simulink library "Simulation_lib"  (R2023a)
settings: Solver=VariableStepAuto  StartTime=0.0  StopTime=10.0  RelTol=1e-3
libraries: $bdroot x14, fl_lib x8, nesl_utility x7, Math x5, ee_lib x3, sdl_lib x2, simulink_extras x1, vrlib x1
settings Model: Creator=FIRSTMentor  LastModifiedBy=FIRSTMentor

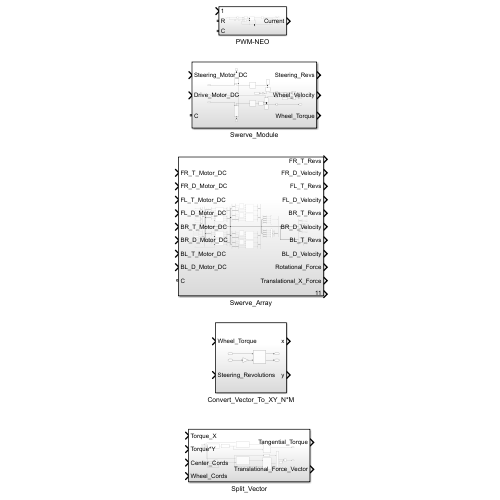
[thumbnail: Simulink's stored preview of the top-level diagram]
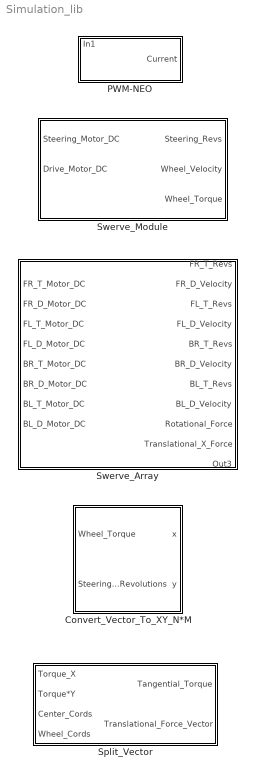
== system Simulation_lib ==
  Convert_Vector_To_XY_N*M : Subsystem
  PWM-NEO : Subsystem
  Split_Vector : Subsystem
  Swerve_Array : Subsystem
  Swerve_Module : Subsystem

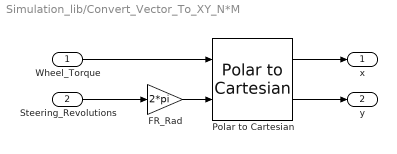
== system Simulation_lib/Convert_Vector_To_XY_N*M ==
  Wheel_Torque : Inport  OutDataTypeStr=double  Unit=N*m
  Steering_Revolutions : Inport  Port=2  OutDataTypeStr=double  Unit=rev  PortDimensions=1
  FR_Rad : Gain  Gain=2*pi
  Polar to Cartesian : simulink_extras/Transformations/Polar to Cartesian
  x : Outport  OutDataTypeStr=double  Unit=N*m  PortDimensions=1
  y : Outport  Port=2  OutDataTypeStr=double  Unit=N*m  PortDimensions=1
  wires:
  Steering_Revolutions/1 -> FR_Rad/1
  FR_Rad/1 -> Polar to Cartesian/2
  Polar to Cartesian/2 -> y/1
  Polar to Cartesian/1 -> x/1
  Wheel_Torque/1 -> Polar to Cartesian/1

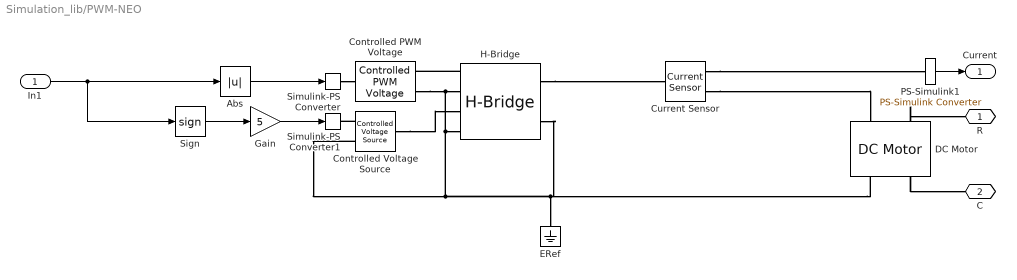
== system Simulation_lib/PWM-NEO ==
  In1 : Inport
  Abs : Abs  SaturateOnIntegerOverflow=off
  Controlled PWM Voltage : ee_lib/Integrated Circuits/Controlled PWM Voltage  F=4000 Hz  TD=0 s  pulse_width_offset=0 s  pulse_min=0 s  pwm_or_av=2  event_type=1  sample_time=5e-6 s  Vmin=0 V  Vmax=5 V  Vm=5 V  u_min=0  u_max=1
      settings: InternalSimscapePortConfiguration="{\"Bottom\":[],\"Left\":[{\"id\":\"u\",\"label\":\"u\",\"type\":\"input\"}],\"Right\":[{\"id\":\"p2\",\"label\":\"PWM\",\"type\":\"foundation.electrical.electrical\"},{\"id\":\"n2\",\"label\":\"REF\",\"type\":\"foundation.electrical.electrical\"}],\"Top\":[]}"
  Controlled Voltage Source : fl_lib/Electrical/Electrical Sources/Controlled Voltage Source
  Current Sensor : fl_lib/Electrical/Electrical Sensors/Current Sensor
  DC Motor : ee_lib/Electromechanical/Brushed Motors/DC Motor  field_option=ee.enum.field_option.pm  Rf=100 Ohm  Lf=1 H  Laf=0.15 H  If0=0 A  parameterization=3  Ra=3.38 Ohm  La=0.01 H  emf_or_torque=1  Kv=0.029 V/(rad/s)  Ki=6.876e-04 N*m/A  T_stall=0.1 N*m  w_max=5700 rpm  w_rated=2910 rpm  P_rated=500 W  V_rated=12 V  lam_param=ee.enum.lam_param.current  i_noload=1.7 A  V_i_noload=12 V  J=0.0002 kg*m^2  lam=0.5e-5 N*m/(rad/s)  speed0=0 rpm  enable_fault_armature=simscape.enum.onoff.off  rev_faulted=1 / 3  G_faulted_armature=1e-5 S  fault_trigger_armature=ee.enum.faults.faultTrigger.temporal  t_fault_armature=1 s  max_permissible_current_armature=inf A  t_fail_on_current_armature=1 s  enable_fault_field=simscape.enum.onoff.off  G_faulted_field=1e-5 S  fault_trigger_field=ee.enum.faults.faultTrigger.temporal  t_fault_field=1 s  max_permissible_current_field=inf A  t_fail_on_current_field=1 s  fault_action=simscape.enum.assert.action.none  alpha=3.93e-3 1/K  Tmeas=25 degC  thermal_mass=100 J/K  initial_temperature=25 degC
  ERef : fl_lib/Electrical/Electrical Elements/Electrical Reference
  Gain : Gain  Gain=5
  H-Bridge : ee_lib/Semiconductors & Converters/Converters/H-Bridge  supply_ports=ee.enum.supply_ports.hidesupply  pwm_or_av=2  regenerative_braking_mode=2  discontinuous=0  freewheeling_mode=1  Rload=3.38+0.1 Ohm  Lload=1e-5 H  F=4 kHz  Venable=2.5 V  Vmax=5 V  Vreverse=2.5 V  Vbrake=2.5 V  Vm=12 V  Ron=0.1 Ohm  Don=0.1 Ohm  Goff=1e-6 S  Tmeas=298.15 K  Ron2=0.1 Ohm  Don2=0.05 Ohm  Tmeas2=398.15 K  thermal_mass=100 J/K  initial_temperature=298.15 K
  PS-Simulink1 : nesl_utility/PS-Simulink Converter  PhysicalDomain=network_engine_domain  SubClassName=ps_output  LeftPortType=input  RightPortType=output  PseudoPeriodic=off  Frequencies=[]  VectorFormat=1-D array  Unit=A  AffineConversion=off
  Sign : Signum
  Simulink-PS Converter : nesl_utility/Simulink-PS Converter  PhysicalDomain=network_engine_domain  SubClassName=ps_input  LeftPortType=input  RightPortType=output  PseudoPeriodic=off  Frequencies=[]  NoiseDistribution=none  NoiseParameters=[]  Unit=1  AffineConversion=off  FilteringAndDerivatives=provide  SimscapeFilterOrder=1  InputFilterTimeConstant=0.001  UdotUserProvided=0
  Simulink-PS Converter1 : nesl_utility/Simulink-PS Converter  PhysicalDomain=network_engine_domain  SubClassName=ps_input  LeftPortType=input  RightPortType=output  PseudoPeriodic=off  Frequencies=[]  NoiseDistribution=none  NoiseParameters=[]  Unit=1  AffineConversion=off  FilteringAndDerivatives=zero  SimscapeFilterOrder=1  InputFilterTimeConstant=0.001  UdotUserProvided=0
  R : PMIOPort  Side=Left
  C : PMIOPort  Port=2  Side=Left
  Current : Outport
  wires:
  PS-Simulink1/1 -> Current/1
  Abs/1 -> Simulink-PS Converter/1
  In1/1 -> Sign/1, Abs/1
  Sign/1 -> Gain/1
  Gain/1 -> Simulink-PS Converter1/1
  connections:
  Current Sensor/RConn1 -- PS-Simulink1/LConn1
  H-Bridge/RConn1 -- Current Sensor/LConn1
  H-Bridge/LConn1 -- Controlled PWM Voltage/RConn1
  Simulink-PS Converter/RConn1 -- Controlled PWM Voltage/LConn1
  DC Motor/RConn2 -- C/RConn1
  DC Motor/LConn2 -- R/RConn1
  Current Sensor/RConn2 -- DC Motor/LConn1
  H-Bridge/LConn4 -- Controlled Voltage Source/RConn2 -- DC Motor/RConn1 -- H-Bridge/RConn2 -- ERef/LConn1 -- H-Bridge/LConn2 -- Controlled PWM Voltage/RConn2
  Controlled Voltage Source/LConn1 -- H-Bridge/LConn3
  Controlled Voltage Source/RConn1 -- Simulink-PS Converter1/RConn1

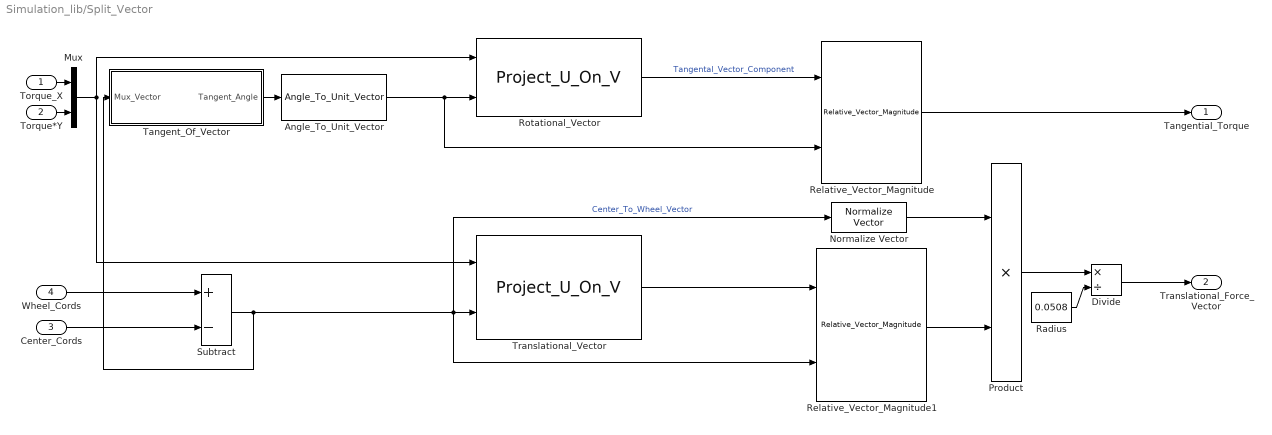
== system Simulation_lib/Split_Vector ==
  Torque_X : Inport  OutDataTypeStr=double  Unit=N*m  PortDimensions=1
  Torque*Y : Inport  Port=2  OutDataTypeStr=double  Unit=N*m  PortDimensions=1
  Center_Cords : Inport  Port=3  OutDataTypeStr=double  Unit=m  PortDimensions=2
  Wheel_Cords : Inport  Port=4  OutDataTypeStr=double  Unit=m  PortDimensions=2
  Angle_To_Unit_Vector : Math/Angle_To_Unit_Vector  SystemSampleTime=-1  VariantActivationTime=update diagram  Latency=0  AutoFrameSizeCalculation=off
  Divide : Product  Inputs=*/
  Mux : Mux  Inputs=2
  Normalize Vector : vrlib/Utilities/Normalize Vector  maxzero=0
  Product : Product
  Radius : Constant  Value=0.0508
  Relative_Vector_Magnitude : Math/Relative_Vector_Magnitude  SystemSampleTime=-1  VariantActivationTime=update diagram  Latency=0  AutoFrameSizeCalculation=off
  Relative_Vector_Magnitude1 : Math/Relative_Vector_Magnitude  SystemSampleTime=-1  VariantActivationTime=update diagram  Latency=0  AutoFrameSizeCalculation=off
  Rotational_Vector : Math/Project_U_On_V  SystemSampleTime=-1  VariantActivationTime=update diagram  Latency=0  AutoFrameSizeCalculation=off
  Subtract : Sum  Inputs=+-
  Tangent_Of_Vector : Subsystem
  Translational_Vector : Math/Project_U_On_V  SystemSampleTime=-1  VariantActivationTime=update diagram  Latency=0  AutoFrameSizeCalculation=off
  Tangential_Torque : Outport  OutDataTypeStr=double  Unit=N*m
  Translational_Force_Vector : Outport  Port=2  OutDataTypeStr=double  Unit=N  PortDimensions=2
  wires:
  Torque_X/1 -> Mux/1
  Torque*Y/1 -> Mux/2
  Mux/1 -> Translational_Vector/1, Rotational_Vector/1
  Tangent_Of_Vector/1(Tangent_Angle) -> Angle_To_Unit_Vector/1
  Center_Cords/1 -> Subtract/2
  Subtract/1 -> Tangent_Of_Vector/1(Mux_Vector), Relative_Vector_Magnitude1/2, Normalize Vector/1, Translational_Vector/2  "Center_To_Wheel_Vector"
  Wheel_Cords/1 -> Subtract/1
  Rotational_Vector/1 -> Relative_Vector_Magnitude/1  "Tangental_Vector_Component"
  Relative_Vector_Magnitude/1 -> Tangential_Torque/1
  Relative_Vector_Magnitude1/1 -> Product/2
  Translational_Vector/1 -> Relative_Vector_Magnitude1/1
  Normalize Vector/1 -> Product/1
  Product/1 -> Divide/1
  Angle_To_Unit_Vector/1 -> Rotational_Vector/2, Relative_Vector_Magnitude/2
  Divide/1 -> Translational_Force_Vector/1
  Radius/1 -> Divide/2

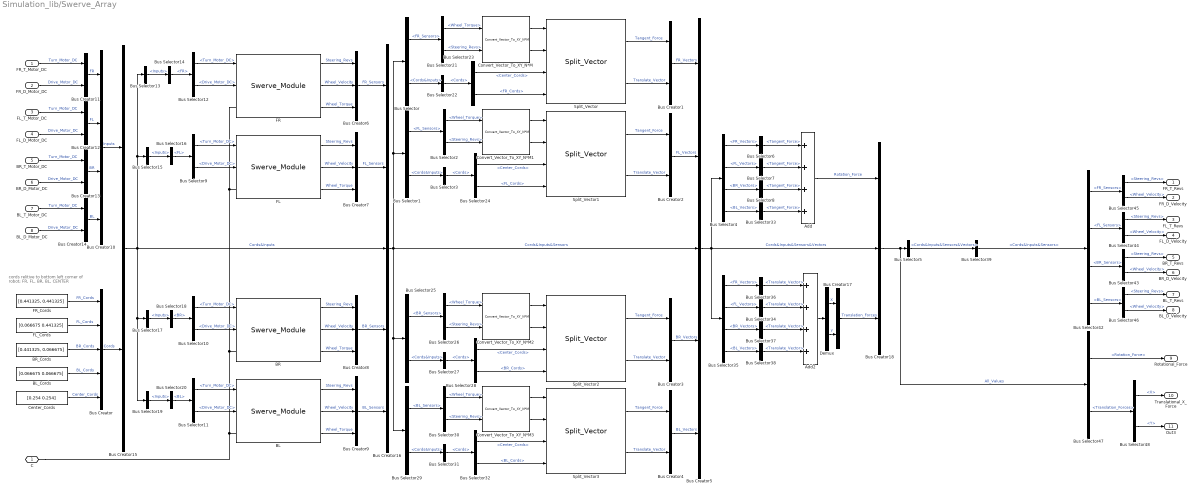
== system Simulation_lib/Swerve_Array ==
  note: cords relitive to bottom left corner of robot; FR, FL, BR, BL, CENTER
  FR_T_Motor_DC : Inport
  FR_D_Motor_DC : Inport  Port=2
  FL_T_Motor_DC : Inport  Port=3
  FL_D_Motor_DC : Inport  Port=4
  BR_T_Motor_DC : Inport  Port=5
  BR_D_Motor_DC : Inport  Port=6
  BL_T_Motor_DC : Inport  Port=7
  BL_D_Motor_DC : Inport  Port=8
  Add : Sum  Inputs=4
  Add2 : Sum  Inputs=4
  BL : $bdroot/Swerve_Module  SystemSampleTime=-1  VariantActivationTime=update diagram  Latency=0  AutoFrameSizeCalculation=off
  BL_Cords : Constant  Value=[0.066675 0.066675]
  BR : $bdroot/Swerve_Module  SystemSampleTime=-1  VariantActivationTime=update diagram  Latency=0  AutoFrameSizeCalculation=off
  BR_Cords : Constant  Value=[0.441325, 0.066675]
  Bus Creator : BusCreator  Inputs=5
  Bus Creator{1..4,11..15,17} (10 alike) : BusCreator  Inputs=2
  Bus Creator10 : BusCreator  Inputs=4
  Bus Creator16 : BusCreator  Inputs=5
  Bus Creator{6..9,18} (5 alike) : BusCreator  Inputs=3
  Bus Creator5 : BusCreator  Inputs=5
  Bus Selector : BusSelector  OutputSignals=FR_Sensors,Cords&Inputs
  Bus Selector1 : BusSelector  OutputSignals=FL_Sensors,Cords&Inputs
  Bus Selector{9..12} (4 alike) : BusSelector  OutputSignals=Turn_Motor_DC,Drive_Motor_DC
  Bus Selector{13,15,17,19} (4 alike) : BusSelector  OutputSignals=Inputs
  Bus Selector14 : BusSelector  OutputSignals=FR
  Bus Selector16 : BusSelector  OutputSignals=FL
  Bus Selector18 : BusSelector  OutputSignals=BR
  Bus Selector{2,21,26,30} (4 alike) : BusSelector  OutputSignals=Wheel_Torque,Steering_Revs
  Bus Selector20 : BusSelector  OutputSignals=BL
  Bus Selector{3,22,27,31} (4 alike) : BusSelector  OutputSignals=Cords
  Bus Selector23 : BusSelector  OutputSignals=Center_Cords,FR_Cords
  Bus Selector24 : BusSelector  OutputSignals=Center_Cords,FL_Cords
  Bus Selector25 : BusSelector  OutputSignals=BR_Sensors,Cords&Inputs
  Bus Selector28 : BusSelector  OutputSignals=Center_Cords,BR_Cords
  Bus Selector29 : BusSelector  OutputSignals=BL_Sensors,Cords&Inputs
  Bus Selector32 : BusSelector  OutputSignals=Center_Cords,BL_Cords
  Bus Selector{6..8,33} (4 alike) : BusSelector  OutputSignals=Tangent_Force
  Bus Selector{34,36..38} (4 alike) : BusSelector  OutputSignals=Translate_Vector
  Bus Selector35 : BusSelector  OutputSignals=FR_Vectors,FL_Vectors,BR_Vectors,BL_Vectors
  Bus Selector39 : BusSelector  OutputSignals=Cords&Inputs&Sensors
  Bus Selector4 : BusSelector  OutputSignals=FR_Vectors,FL_Vectors,BR_Vectors,BL_Vectors
  Bus Selector42 : BusSelector  OutputSignals=FR_Sensors,FL_Sensors,BR_Sensors,BL_Sensors
  Bus Selector{43..46} (4 alike) : BusSelector  OutputSignals=Steering_Revs,Wheel_Velocity
  Bus Selector47 : BusSelector  OutputSignals=Rotation_Force,Translation_Forces
  Bus Selector48 : BusSelector  OutputSignals=X,Y
  Bus Selector5 : BusSelector  OutputSignals=Cords&Inputs&Sensors&Vectors
  Center_Cords : Constant  Value=[0.254 0.254]
  Convert_Vector_To_XY_N*M{,1..3} (4 alike) : $bdroot/Convert_Vector_To_XY_N*M  SystemSampleTime=-1  VariantActivationTime=update diagram  Latency=0  AutoFrameSizeCalculation=off
  Demux : Demux  Outputs=2
  FL : $bdroot/Swerve_Module  SystemSampleTime=-1  VariantActivationTime=update diagram  Latency=0  AutoFrameSizeCalculation=off
  FL_Cords : Constant  Value=[0.066675 0.441325]
  FR : $bdroot/Swerve_Module  SystemSampleTime=-1  VariantActivationTime=update diagram  Latency=0  AutoFrameSizeCalculation=off
  FR_Cords : Constant  Value=[0.441325, 0.441325]
  Split_Vector{,1..3} (4 alike) : $bdroot/Split_Vector  SystemSampleTime=-1  VariantActivationTime=update diagram  Latency=0  AutoFrameSizeCalculation=off
  C : PMIOPort  Side=Left
  FR_T_Revs : Outport
  FR_D_Velocity : Outport  Port=2
  FL_T_Revs : Outport  Port=3
  FL_D_Velocity : Outport  Port=4
  BR_T_Revs : Outport  Port=5
  BR_D_Velocity : Outport  Port=6
  BL_T_Revs : Outport  Port=7
  BL_D_Velocity : Outport  Port=8
  Rotational_Force : Outport  Port=9
  Translational_X_Force : Outport  Port=10
  Out3 : Outport  Port=11
  wires:
  FR_Cords/1 -> Bus Creator/1  "FR_Cords"
  FL_Cords/1 -> Bus Creator/2  "FL_Cords"
  BR_Cords/1 -> Bus Creator/3  "BR_Cords"
  BL_Cords/1 -> Bus Creator/4  "BL_Cords"
  Center_Cords/1 -> Bus Creator/5  "Center_Cords"
  Convert_Vector_To_XY_N*M/1 -> Split_Vector/1
  Convert_Vector_To_XY_N*M/2 -> Split_Vector/2
  Convert_Vector_To_XY_N*M1/1 -> Split_Vector1/1
  Convert_Vector_To_XY_N*M1/2 -> Split_Vector1/2
  Convert_Vector_To_XY_N*M2/1 -> Split_Vector2/1
  Convert_Vector_To_XY_N*M2/2 -> Split_Vector2/2
  Convert_Vector_To_XY_N*M3/1 -> Split_Vector3/1
  Convert_Vector_To_XY_N*M3/2 -> Split_Vector3/2
  Split_Vector/1 -> Bus Creator1/1  "Tangent_Force"
  Split_Vector/2 -> Bus Creator1/2  "Translate_Vector"
  Split_Vector1/2 -> Bus Creator2/2  "Translate_Vector"
  Split_Vector1/1 -> Bus Creator2/1  "Tangent_Force"
  Split_Vector2/1 -> Bus Creator3/1  "Tangent_Force"
  Split_Vector2/2 -> Bus Creator3/2  "Translate_Vector"
  Split_Vector3/2 -> Bus Creator4/2  "Translate_Vector"
  Split_Vector3/1 -> Bus Creator4/1  "Tangent_Force"
  Bus Creator1/1 -> Bus Creator5/1  "FR_Vectors"
  Bus Creator2/1 -> Bus Creator5/2  "FL_Vectors"
  Bus Creator3/1 -> Bus Creator5/4  "BR_Vectors"
  Bus Creator4/1 -> Bus Creator5/5  "BL_Vectors"
  FR/2 -> Bus Creator6/2  "Wheel_Velocity"
  FR/1 -> Bus Creator6/1  "Steering_Revs"
  FR/3 -> Bus Creator6/3  "Wheel_Torque"
  FL/1 -> Bus Creator7/1  "Steering_Revs"
  FL/2 -> Bus Creator7/2  "Wheel_Velocity"
  FL/3 -> Bus Creator7/3  "Wheel_Torque"
  BL/1 -> Bus Creator9/1  "Steering_Revs"
  BL/2 -> Bus Creator9/2  "Wheel_Velocity"
  BL/3 -> Bus Creator9/3  "Wheel_Torque"
  BR/3 -> Bus Creator8/3  "Wheel_Torque"
  BR/2 -> Bus Creator8/2  "Wheel_Velocity"
  BR/1 -> Bus Creator8/1  "Steering_Revs"
  FR_T_Motor_DC/1 -> Bus Creator11/1  "Turn_Motor_DC"
  FR_D_Motor_DC/1 -> Bus Creator11/2  "Drive_Motor_DC"
  FL_T_Motor_DC/1 -> Bus Creator12/1  "Turn_Motor_DC"
  FL_D_Motor_DC/1 -> Bus Creator12/2  "Drive_Motor_DC"
  BR_T_Motor_DC/1 -> Bus Creator13/1  "Turn_Motor_DC"
  BR_D_Motor_DC/1 -> Bus Creator13/2  "Drive_Motor_DC"
  BL_T_Motor_DC/1 -> Bus Creator14/1  "Turn_Motor_DC"
  BL_D_Motor_DC/1 -> Bus Creator14/2  "Drive_Motor_DC"
  Bus Creator12/1 -> Bus Creator10/2  "FL"
  Bus Creator11/1 -> Bus Creator10/1  "FR"
  Bus Creator13/1 -> Bus Creator10/3  "BR"
  Bus Creator14/1 -> Bus Creator10/4  "BL"
  Bus Creator10/1 -> Bus Creator15/1  "Inputs"
  Bus Creator/1 -> Bus Creator15/2  "Cords"
  Bus Creator15/1 -> Bus Selector19/1, Bus Selector17/1, Bus Creator16/3, Bus Selector13/1, Bus Selector15/1  "Cords&Inputs"
  Bus Selector9/1 -> FL/1  "<Turn_Motor_DC>"
  Bus Selector9/2 -> FL/2  "<Drive_Motor_DC>"
  Bus Selector10/1 -> BR/1  "<Turn_Motor_DC>"
  Bus Selector10/2 -> BR/2  "<Drive_Motor_DC>"
  Bus Selector11/1 -> BL/1  "<Turn_Motor_DC>"
  Bus Selector11/2 -> BL/2  "<Drive_Motor_DC>"
  Bus Selector12/1 -> FR/1  "<Turn_Motor_DC>"
  Bus Selector12/2 -> FR/2  "<Drive_Motor_DC>"
  Bus Selector13/1 -> Bus Selector14/1  "<Inputs>"
  Bus Selector14/1 -> Bus Selector12/1  "<FR>"
  Bus Selector15/1 -> Bus Selector16/1  "<Inputs>"
  Bus Selector16/1 -> Bus Selector9/1  "<FL>"
  Bus Selector17/1 -> Bus Selector18/1  "<Inputs>"
  Bus Selector18/1 -> Bus Selector10/1  "<BR>"
  Bus Selector19/1 -> Bus Selector20/1  "<Inputs>"
  Bus Selector20/1 -> Bus Selector11/1  "<BL>"
  Bus Creator6/1 -> Bus Creator16/1  "FR_Sensors"
  Bus Creator7/1 -> Bus Creator16/2  "FL_Sensors"
  Bus Creator9/1 -> Bus Creator16/5  "BL_Sensors"
  Bus Creator8/1 -> Bus Creator16/4  "BR_Sensors"
  Bus Creator16/1 -> Bus Selector/1, Bus Selector1/1, Bus Creator5/3, Bus Selector29/1, Bus Selector25/1  "Cords&Inputs&Sensors"
  Bus Selector/1 -> Bus Selector21/1  "<FR_Sensors>"
  Bus Selector21/1 -> Convert_Vector_To_XY_N*M/1  "<Wheel_Torque>"
  Bus Selector21/2 -> Convert_Vector_To_XY_N*M/2  "<Steering_Revs>"
  Bus Selector/2 -> Bus Selector22/1  "<Cords&Inputs>"
  Bus Selector22/1 -> Bus Selector23/1  "<Cords>"
  Bus Selector23/1 -> Split_Vector/3  "<Center_Cords>"
  Bus Selector23/2 -> Split_Vector/4  "<FR_Cords>"
  Bus Selector2/1 -> Convert_Vector_To_XY_N*M1/1  "<Wheel_Torque>"
  Bus Selector3/1 -> Bus Selector24/1  "<Cords>"
  Bus Selector24/2 -> Split_Vector1/4  "<FL_Cords>"
  Bus Selector1/2 -> Bus Selector3/1  "<Cords&Inputs>"
  Bus Selector1/1 -> Bus Selector2/1  "<FL_Sensors>"
  Bus Selector2/2 -> Convert_Vector_To_XY_N*M1/2  "<Steering_Revs>"
  Bus Selector24/1 -> Split_Vector1/3  "<Center_Cords>"
  Bus Selector26/1 -> Convert_Vector_To_XY_N*M2/1  "<Wheel_Torque>"
  Bus Selector27/1 -> Bus Selector28/1  "<Cords>"
  Bus Selector28/2 -> Split_Vector2/4  "<BR_Cords>"
  Bus Selector25/2 -> Bus Selector27/1  "<Cords&Inputs>"
  Bus Selector25/1 -> Bus Selector26/1  "<BR_Sensors>"
  Bus Selector26/2 -> Convert_Vector_To_XY_N*M2/2  "<Steering_Revs>"
  Bus Selector28/1 -> Split_Vector2/3  "<Center_Cords>"
  Bus Selector30/1 -> Convert_Vector_To_XY_N*M3/1  "<Wheel_Torque>"
  Bus Selector31/1 -> Bus Selector32/1  "<Cords>"
  Bus Selector32/2 -> Split_Vector3/4  "<BL_Cords>"
  Bus Selector29/2 -> Bus Selector31/1  "<Cords&Inputs>"
  Bus Selector29/1 -> Bus Selector30/1  "<BL_Sensors>"
  Bus Selector30/2 -> Convert_Vector_To_XY_N*M3/2  "<Steering_Revs>"
  Bus Selector32/1 -> Split_Vector3/3  "<Center_Cords>"
  Bus Selector4/1 -> Bus Selector6/1  "<FR_Vectors>"
  Bus Selector4/2 -> Bus Selector7/1  "<FL_Vectors>"
  Bus Selector4/3 -> Bus Selector8/1  "<BR_Vectors>"
  Bus Selector4/4 -> Bus Selector33/1  "<BL_Vectors>"
  Bus Selector6/1 -> Add/1  "<Tangent_Force>"
  Bus Selector7/1 -> Add/2  "<Tangent_Force>"
  Bus Selector8/1 -> Add/3  "<Tangent_Force>"
  Bus Selector33/1 -> Add/4  "<Tangent_Force>"
  Add/1 -> Bus Creator18/1  "Rotation_Force"
  Bus Creator5/1 -> Bus Selector4/1, Bus Creator18/2, Bus Selector35/1  "Cords&Inputs&Sensors&Vectors"
  Bus Selector38/1 -> Add2/4  "<Translate_Vector>"
  Bus Selector35/4 -> Bus Selector38/1  "<BL_Vectors>"
  Demux/1 -> Bus Creator17/1  "X"
  Bus Selector34/1 -> Add2/2  "<Translate_Vector>"
  Demux/2 -> Bus Creator17/2  "Y"
  Add2/1 -> Demux/1
  Bus Selector35/3 -> Bus Selector37/1  "<BR_Vectors>"
  Bus Selector35/2 -> Bus Selector34/1  "<FL_Vectors>"
  Bus Selector37/1 -> Add2/3  "<Translate_Vector>"
  Bus Selector36/1 -> Add2/1  "<Translate_Vector>"
  Bus Selector35/1 -> Bus Selector36/1  "<FR_Vectors>"
  Bus Creator17/1 -> Bus Creator18/3  "Translation_Forces"
  Bus Creator18/1 -> Bus Selector5/1, Bus Selector47/1  "All_Values"
  Bus Selector5/1 -> Bus Selector39/1  "<Cords&Inputs&Sensors&Vectors>"
  Bus Selector39/1 -> Bus Selector42/1  "<Cords&Inputs&Sensors>"
  Bus Selector42/4 -> Bus Selector46/1  "<BL_Sensors>"
  Bus Selector46/1 -> BL_T_Revs/1  "<Steering_Revs>"
  Bus Selector46/2 -> BL_D_Velocity/1  "<Wheel_Velocity>"
  Bus Selector43/1 -> BR_T_Revs/1  "<Steering_Revs>"
  Bus Selector43/2 -> BR_D_Velocity/1  "<Wheel_Velocity>"
  Bus Selector42/3 -> Bus Selector43/1  "<BR_Sensors>"
  Bus Selector44/1 -> FL_T_Revs/1  "<Steering_Revs>"
  Bus Selector44/2 -> FL_D_Velocity/1  "<Wheel_Velocity>"
  Bus Selector42/2 -> Bus Selector44/1  "<FL_Sensors>"
  Bus Selector45/1 -> FR_T_Revs/1  "<Steering_Revs>"
  Bus Selector45/2 -> FR_D_Velocity/1  "<Wheel_Velocity>"
  Bus Selector42/1 -> Bus Selector45/1  "<FR_Sensors>"
  Bus Selector47/1 -> Rotational_Force/1  "<Rotation_Force>"
  Bus Selector47/2 -> Bus Selector48/1  "<Translation_Forces>"
  Bus Selector48/2 -> Out3/1  "<Y>"
  Bus Selector48/1 -> Translational_X_Force/1  "<X>"
  connections:
  BR/LConn1 -- C/RConn1 -- BL/LConn1 -- FR/LConn1 -- FL/LConn1

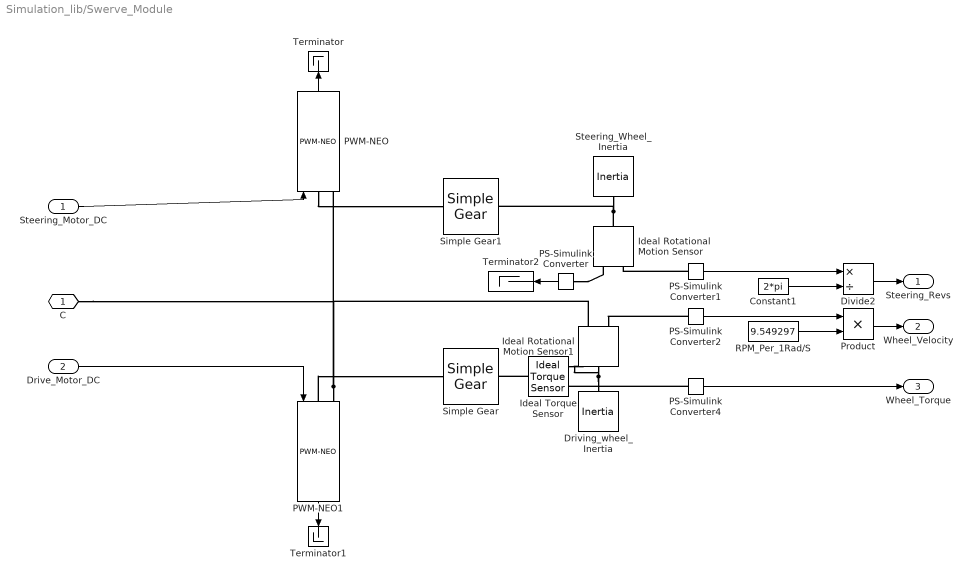
== system Simulation_lib/Swerve_Module ==
  Steering_Motor_DC : Inport
  Drive_Motor_DC : Inport  Port=2
  Constant1 : Constant  Value=2*pi
  Divide2 : Product  Inputs=*/
  Driving_wheel_Inertia : fl_lib/Mechanical/Rotational Elements/Inertia  inertia=1.315 lbm*in^2  num_ports=foundation.enum.numPorts2.one  w_specify=off  w_priority=High  w=0 rad/s  w_nominal_specify=off  w_nominal_unit=rad/s  w_nominal_value=1  t_specify=off  t_priority=None  t=0 N*m  t_nominal_specify=off  t_nominal_unit=N*m  t_nominal_value=1
  Ideal Rotational Motion Sensor : fl_lib/Mechanical/Mechanical Sensors/Ideal Rotational Motion Sensor  reference=foundation.enum.MeasurementReference.absolute  acceleration_port=false  velocity_port=true  position_port=true  wrap_angle=false  offset=0 rad
      settings: InternalSimscapePortConfiguration="{\"Bottom\":[],\"Left\":[{\"id\":\"R\",\"label\":\"R\",\"type\":\"foundation.mechanical.rotational.rotational\"}],\"Right\":[{\"id\":\"W\",\"label\":\"W\",\"type\":\"output\"},{\"id\":\"A\",\"label\":\"A\",\"type\":\"output\"}],\"Top\":[]}"
  Ideal Rotational Motion Sensor1 : fl_lib/Mechanical/Mechanical Sensors/Ideal Rotational Motion Sensor  reference=foundation.enum.MeasurementReference.difference  acceleration_port=false  velocity_port=true  position_port=false  wrap_angle=false  offset=0 rad
      settings: InternalSimscapePortConfiguration="{\"Bottom\":[],\"Left\":[{\"id\":\"R\",\"label\":\"R\",\"type\":\"foundation.mechanical.rotational.rotational\"}],\"Right\":[{\"id\":\"C\",\"label\":\"C\",\"type\":\"foundation.mechanical.rotational.rotational\"},{\"id\":\"W\",\"label\":\"W\",\"type\":\"output\"}],\"Top\":[]}"
  Ideal Torque Sensor : fl_lib/Mechanical/Mechanical Sensors/Ideal Torque Sensor
  PS-Simulink Converter : nesl_utility/PS-Simulink Converter  PhysicalDomain=network_engine_domain  SubClassName=ps_output  LeftPortType=input  RightPortType=output  PseudoPeriodic=off  Frequencies=[]  VectorFormat=inherit  Unit=inherit  AffineConversion=off
  PS-Simulink Converter1 : nesl_utility/PS-Simulink Converter  PhysicalDomain=network_engine_domain  SubClassName=ps_output  LeftPortType=input  RightPortType=output  PseudoPeriodic=off  Frequencies=[]  VectorFormat=inherit  Unit=inherit  AffineConversion=off
  PS-Simulink Converter2 : nesl_utility/PS-Simulink Converter  PhysicalDomain=network_engine_domain  SubClassName=ps_output  LeftPortType=input  RightPortType=output  PseudoPeriodic=off  Frequencies=[]  VectorFormat=inherit  Unit=rad/s  AffineConversion=off
  PS-Simulink Converter4 : nesl_utility/PS-Simulink Converter  PhysicalDomain=network_engine_domain  SubClassName=ps_output  LeftPortType=input  RightPortType=output  PseudoPeriodic=off  Frequencies=[]  VectorFormat=inherit  Unit=inherit  AffineConversion=off
  PWM-NEO : $bdroot/PWM-NEO  SystemSampleTime=-1  VariantActivationTime=update diagram  Latency=0  AutoFrameSizeCalculation=off
  PWM-NEO1 : $bdroot/PWM-NEO  SystemSampleTime=-1  VariantActivationTime=update diagram  Latency=0  AutoFrameSizeCalculation=off
  Product : Product
  RPM_Per_1Rad/S : Constant  Value=9.549297
  Simple Gear : sdl_lib/Gears/Simple Gear  ratio=8.14  rotation_direction=sdl.enum.shaftOutputDirection.opposite  friction_model=sdl.enum.gear_efficiencies_load.off  T_noload=0.1 N*m  T_nom=5 N*m  efficiency_nom=0.8  efficiency=0.8  temperature_TLU=[280, 300, 320] K  load_TLU=[1, 5, 10] N*m  efficiency_TLU=[.95, .9, .85]  efficiency_TLU2=[.85, .8, .75; .95, .9, .85; .85, .8, .7]  w_thr=0.01 rad/s  pwr_thr=0.001 W  enable_backlash=false  hardstop_model=simscape.enum.hardstop.smooth  backlash_distance=1e-3 mm  r_base=0.1 m  transition=1e-4 mm  backlash_stiffness=1e6 N/m  backlash_damping=1e3 N*s/m  coeff_rest=0.7  v_tol=0.001 m/s  f_tol=0.001 N  mu_visc=[0, 0] N*m*s/rad  enable_faults=simscape.enum.onoff.off  efficiency_fault=0.05  external_fault=simscape.enum.onoff.off  temporal_fault=simscape.enum.onoff.off  fault_time=5 s  fault_angles=pi / 12 rad  report_fault=simscape.enum.assert.action.none  thermal_mass=50 J/K  temperature_specify=off  temperature_priority=High  temperature=300 K  temperature_nominal_specify=off  temperature_nominal_unit=K  temperature_nominal_value=1  x_backlash_specify=off  x_backlash_priority=None  x_backlash=0 mm  x_backlash_nominal_specify=off  x_backlash_nominal_unit=mm  x_backlash_nominal_value=1  f_hardstop_specify=off  f_hardstop_priority=None  f_hardstop=0 N  f_hardstop_nominal_specify=off  f_hardstop_nominal_unit=N  f_hardstop_nominal_value=1  v_backlash_specify=off  v_backlash_priority=None  v_backlash=0 m/s  v_backlash_nominal_specify=off  v_backlash_nominal_unit=m/s  v_backlash_nominal_value=1
  Simple Gear1 : sdl_lib/Gears/Simple Gear  ratio=150/7  rotation_direction=sdl.enum.shaftOutputDirection.opposite  friction_model=sdl.enum.gear_efficiencies_load.off  T_noload=0.1 N*m  T_nom=5 N*m  efficiency_nom=0.8  efficiency=0.8  temperature_TLU=[280, 300, 320] K  load_TLU=[1, 5, 10] N*m  efficiency_TLU=[.95, .9, .85]  efficiency_TLU2=[.85, .8, .75; .95, .9, .85; .85, .8, .7]  w_thr=0.01 rad/s  pwr_thr=0.001 W  enable_backlash=false  hardstop_model=simscape.enum.hardstop.smooth  backlash_distance=1e-3 mm  r_base=0.1 m  transition=1e-4 mm  backlash_stiffness=1e6 N/m  backlash_damping=1e3 N*s/m  coeff_rest=0.7  v_tol=0.001 m/s  f_tol=0.001 N  mu_visc=[0, 0] N*m*s/rad  enable_faults=simscape.enum.onoff.off  efficiency_fault=0.05  external_fault=simscape.enum.onoff.off  temporal_fault=simscape.enum.onoff.off  fault_time=5 s  fault_angles=pi / 12 rad  report_fault=simscape.enum.assert.action.none  thermal_mass=50 J/K  temperature_specify=off  temperature_priority=High  temperature=300 K  temperature_nominal_specify=off  temperature_nominal_unit=K  temperature_nominal_value=1  x_backlash_specify=off  x_backlash_priority=None  x_backlash=0 mm  x_backlash_nominal_specify=off  x_backlash_nominal_unit=mm  x_backlash_nominal_value=1  f_hardstop_specify=off  f_hardstop_priority=None  f_hardstop=0 N  f_hardstop_nominal_specify=off  f_hardstop_nominal_unit=N  f_hardstop_nominal_value=1  v_backlash_specify=off  v_backlash_priority=None  v_backlash=0 m/s  v_backlash_nominal_specify=off  v_backlash_nominal_unit=m/s  v_backlash_nominal_value=1
  Steering_Wheel_Inertia : fl_lib/Mechanical/Rotational Elements/Inertia  inertia=2.456 lbm*in^2  num_ports=foundation.enum.numPorts2.one  w_specify=off  w_priority=High  w=0 rad/s  w_nominal_specify=off  w_nominal_unit=rad/s  w_nominal_value=1  t_specify=off  t_priority=None  t=0 N*m  t_nominal_specify=off  t_nominal_unit=N*m  t_nominal_value=1
  Terminator : Terminator
  Terminator1 : Terminator
  Terminator2 : Terminator
  C : PMIOPort  Side=Left
  Steering_Revs : Outport
  Wheel_Velocity : Outport  Port=2  OutDataTypeStr=double  Unit=rpm  PortDimensions=1
  Wheel_Torque : Outport  Port=3  Unit=N*m  PortDimensions=1
  wires:
  Divide2/1 -> Steering_Revs/1
  Product/1 -> Wheel_Velocity/1
  Drive_Motor_DC/1 -> PWM-NEO1/1
  Steering_Motor_DC/1 -> PWM-NEO/1
  RPM_Per_1Rad/S/1 -> Product/2
  PS-Simulink Converter1/1 -> Divide2/1
  Constant1/1 -> Divide2/2
  PS-Simulink Converter2/1 -> Product/1
  PWM-NEO1/1 -> Terminator1/1
  PWM-NEO/1 -> Terminator/1
  PS-Simulink Converter4/1 -> Wheel_Torque/1
  PS-Simulink Converter/1 -> Terminator2/1
  connections:
  Ideal Torque Sensor/LConn1 -- Simple Gear/RConn1
  PWM-NEO1/LConn2 -- C/RConn1 -- PWM-NEO/LConn2 -- Ideal Rotational Motion Sensor1/RConn1
  PWM-NEO1/LConn1 -- Simple Gear/LConn1
  Ideal Rotational Motion Sensor/LConn1 -- Simple Gear1/RConn1 -- Steering_Wheel_Inertia/LConn1
  Ideal Torque Sensor/RConn1 -- Driving_wheel_Inertia/LConn1 -- Ideal Rotational Motion Sensor1/LConn1
  PS-Simulink Converter2/LConn1 -- Ideal Rotational Motion Sensor1/RConn2
  PS-Simulink Converter1/LConn1 -- Ideal Rotational Motion Sensor/RConn2
  PWM-NEO/LConn1 -- Simple Gear1/LConn1
  PS-Simulink Converter4/LConn1 -- Ideal Torque Sensor/RConn2
  PS-Simulink Converter/LConn1 -- Ideal Rotational Motion Sensor/RConn1

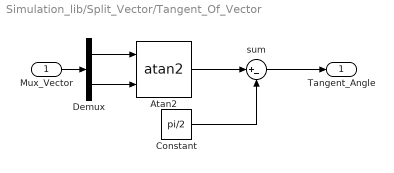
== system Simulation_lib/Split_Vector/Tangent_Of_Vector ==
  Mux_Vector : Inport
  Atan2 : Trigonometry  Operator=atan2
  Constant : Constant  Value=pi/2
  Demux : Demux  Outputs=2
  sum : Sum  Inputs=|+-
  Tangent_Angle : Outport
  wires:
  Demux/1 -> Atan2/1
  Mux_Vector/1 -> Demux/1
  Demux/2 -> Atan2/2
  Atan2/1 -> sum/1
  Constant/1 -> sum/2
  sum/1 -> Tangent_Angle/1
